simulink model "Final_simulation"  (R2024b)
settings: Solver=VariableStepAuto  StartTime=0  StopTime=5*4  FixedStep=1e-6  RelTol=1e-3
libraries: fl_lib x16, spsSeriesRLCBranchLib x9, nesl_utility x8, spsDiodeLib x6, spsMosfetLib x4, spsPWMGeneratorDCDCLib x4, spsControlledVoltageSourceLib x3, slpidlib x2, spsVoltageMeasurementLib x2, spsDCMachineLib x1, spsDCVoltageSourceLib x1, spsGroundLib x1
settings Model: SimulationMode=accelerator  Creator=06MBC93  LastModifiedBy=kamer
settings RTWCC: GPUComputeCapability=3.5

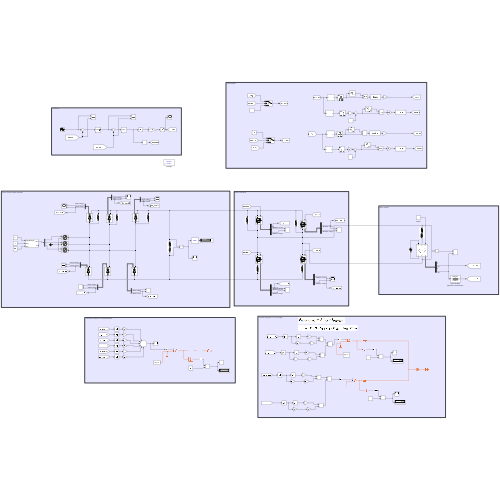
[thumbnail: Simulink's stored preview of the top-level diagram]
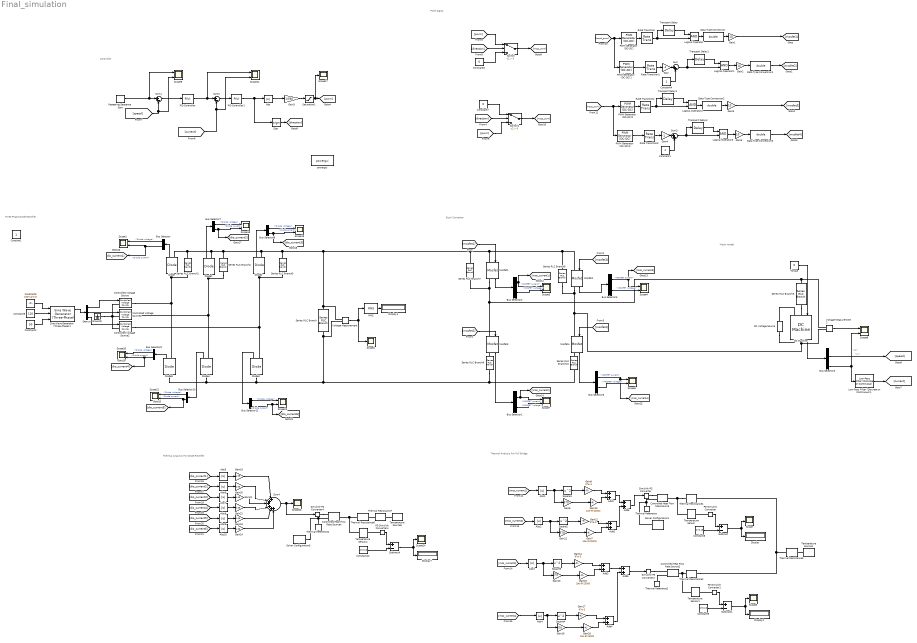
== system Final_simulation ==
  note: Thermal Analysis For Diode Rectifier
  note: Thermal Analysis For Full Bridge
  note: Three Phase Diode Rectifier
  note: Motor model
  note: Buck Converter
  note: PWM Signal
  note: Controller
  Abs{,1..10} (11 alike) : Abs  SaturateOnIntegerOverflow=off
  Add{1..6} (6 alike) : Sum
  Bus Selector{,7..11} (6 alike) : BusSelector  OutputSignals=Diode voltage,Diode current
  Bus Selector{1..2,5..6} (4 alike) : BusSelector  OutputSignals=MOSFET current,MOSFET voltage
  Bus Selector3 : BusSelector  OutputSignals=Te,w,iF,iA
  Constant1 : Constant
  Constant12 : Constant  Value=273.15
  Constant2 : Constant  Value=50
  Constant3 : Constant  Value=230*sqrt(2)
  Constant4 : Constant
  Constant5 : Constant  Value=120
  Constant6 : Constant  Value=0
  Constant7 : Constant  Value=0
  Constant8 : Constant  Value=273.15
  Constant9 : Constant  Value=273.15
  Controlled Heat Flow Rate Source : fl_lib/Thermal/Thermal Sources/Controlled Heat Flow Rate Source
  Controlled Heat Flow Rate Source2 : fl_lib/Thermal/Thermal Sources/Controlled Heat Flow Rate Source
  Controlled Heat Flow Rate Source4 : fl_lib/Thermal/Thermal Sources/Controlled Heat Flow Rate Source
  Controlled Voltage Source : spsControlledVoltageSourceLib/Controlled Voltage Source  Initialize=on  Source_Type=DC  Amplitude=0  Phase=0  Frequency=50  Measurements=None
  Controlled Voltage Source1 : spsControlledVoltageSourceLib/Controlled Voltage Source  Initialize=on  Source_Type=DC  Amplitude=0  Phase=120  Frequency=50  Measurements=None
  Controlled Voltage Source2 : spsControlledVoltageSourceLib/Controlled Voltage Source  Initialize=on  Source_Type=DC  Amplitude=0  Phase=240  Frequency=50  Measurements=None
  DC Machine : spsDCMachineLib/DC Machine  PresetModel=No  MechanicalLoad=Torque TL  FieldType=Wound  ShowDetailedParameters=on  MeasurementBus=on  RLa="[ 0.8  0.0125]"  RLf="[ 210  23]"  Laf=0.482  MachineConstant=Torque constant (N.m/A)  Ke=1.8  Kt=1.8  J=0.12  Bm=0.03  Tf=0.13  w0=0  Ifinit=1.04761904756944  TsPowergui=0  TsBlock=-1
  DC Voltage Source : spsDCVoltageSourceLib/DC Voltage Source  Amplitude=220  Measurements=None
  Data Type Conversion{,1..3} (4 alike) : DataTypeConversion  OutDataTypeStr=double  SaturateOnIntegerOverflow=off  RndMeth=Floor
  Demux : Demux  Outputs=3
  Diode{,1..5} (6 alike) : spsDiodeLib/Diode  Ron=0.015  Lon=0  Vf=1.05  IC=0  UseSnubber=0  Rs=inf  Cs=0  Measurements=on
  Display{,1..2,7} (4 alike) : Display
  Gain : Gain  Gain=-1
  Gain{1..2,5..6} (4 alike) : Gain  Gain=10
  Gain{7,10,15,18} (4 alike) : Gain  Gain=10e-9*25000
  Gain{8,11,13,16} (4 alike) : Gain  Gain=570
  Gain{9,12,14,17} (4 alike) : Gain  Gain=97e-3
  Gain{19..24} (6 alike) : Gain  Gain=1.05
  Gain3 : Gain  Gain=1/560
  Gain4 : Gain  Gain=-1
  Ground1 : spsGroundLib/Ground  LConnTagsString=a
  Logical Operator{,1..3} (4 alike) : Logic  AllPortsSameDT=off  OutDataTypeStr=boolean
  Low-Pass Filter (Discrete or Continuous)1 : eeGeneralControl/Low-Pass Filter (Discrete or Continuous)  K=1  T=0.008  B=inf  A=-inf  init_option=Inherited from block input  x0=0  Ts=-1
  Mosfet{1..4} (4 alike) : spsMosfetLib/Mosfet  Ron=97e-3*1.4  Lon=0  Rd=0.01  Vfd=1.6  IC=0  Rs=inf  Cs=0  Measurements=on
  PID Controller : slpidlib/PID Controller  Controller=PI  Form=Parallel  TimeDomain=Discrete-time  UseExternalTs=off  SampleTime=1/1000  IntegratorMethod=Forward Euler  FilterMethod=Forward Euler  ControllerParametersSource=internal  P=15  I=0.15  UseKiTs=on  D=0.001  UseExternalDerivativeSource=off  N=100  UseFilter=on  TunerSelectOption=Transfer Function Based (PID Tuner App)  InitialConditionSource=internal  InitialConditionForIntegrator=0  InitialConditionForFilter=0  DifferentiatorICPrevScaledInput=0  ExternalReset=none  TrackingMode=off  Kt=1  LimitOutput=on  SatLimitsSource=internal  UpperSaturationLimit=15  LowerSaturationLimit=-15  LinearizeAsGain=on  AntiWindupMode=clamping  Kb=1  LimitIntegrator=off  UpperIntegratorSaturationLimit=inf  LowerIntegratorSaturationLimit=-inf  POutMin=[]  POutMax=[]  IOutMin=[]  IOutMax=[]  DOutMin=[]  DOutMax=[]  NOutMin=[]  NOutMax=[]  SumOutMin=[]  SumOutMax=[]  SaturationOutMin=[]  SaturationOutMax=[]  PParamMin=[]  PParamMax=[]  IParamMin=[]  IParamMax=[]  DParamMin=[]  DParamMax=[]  NParamMin=[]  NParamMax=[]  KbParamMin=[]  KbParamMax=[]  KtParamMin=[]  KtParamMax=[]  KbOutMin=[]  KbOutMax=[]  KtOutMin=[]  KtOutMax=[]  IntegratorOutMin=[]  IntegratorOutMax=[]  FilterOutMin=[]  FilterOutMax=[]  SumI1OutMin=[]  SumI1OutMax=[]  SumI2OutMin=[]  SumI2OutMax=[]  SumI3OutMin=[]  SumI3OutMax=[]  SumI4OutMin=[]  SumI4OutMax=[]  SumDOutMin=[]  SumDOutMax=[]  DifferentiatorOutMin=[]  DifferentiatorOutMax=[]  FilterDiffOutCoefMin=[]  FilterDiffOutCoefMax=[]  ReciprocalOutMin=[]  ReciprocalOutMax=[]  SumDenOutMin=[]  SumDenOutMax=[]  SumNumOutMin=[]  SumNumOutMax=[]  DivideOutMin=[]  DivideOutMax=[]  UdiffTsProdOutMin=[]  UdiffTsProdOutMax=[]  NTsProdOutMin=[]  NTsProdOutMax=[]  UintegralTsProdOutMin=[]  UintegralTsProdOutMax=[]  UngainTsProdOutMin=[]  UngainTsProdOutMax=[]  ClampingZeroOutDataTypeStr=Inherit: Inherit via back propagation  ClampingZeroOutMin=[]  ClampingZeroOutMax=[]  FilterDenConstantOutDataTypeStr=Inherit: Inherit via back propagation  FilterDenConstantOutMin=[]  FilterDenConstantOutMax=[]  PCopyOutDataTypeStr=Inherit: Inherit via back propagation  PCopyOutMin=[]  PCopyOutMax=[]  NCopyOutDataTypeStr=Inherit: Inherit via back propagation  NCopyOutMin=[]  NCopyOutMax=[]  IntegratorContinuousStateAttributes=''  IntegratorStateMustResolveToSignalObject=off  IntegratorRTWStateStorageClass=Auto  FilterContinuousStateAttributes=''  FilterStateMustResolveToSignalObject=off  FilterRTWStateStorageClass=Auto  ParallelPVariant=InternalParameters  IdealPVariant=Disabled  IVariant=InternalParameters  DVariant=Disabled  IntegratorVariant=Discrete  SatVariant=Enabled  AWVariant=DiscClampingParallel  PCopyVariant=Disabled  TRVariant=Disabled  FdbkBlocksVariant=Forward  IdealPFdbkVariant=Disabled  SatFdbkVariant=Disabled  DerivativeFilterVariant=Disabled  NVariant=Disabled  NCopyVariant=Disabled_SignalSpec  FilterICVariant=Disabled  IntegratorICVariant=InternalICs  ExternalResetVariant=Disabled  TRSumVariant=Passthrough  SumFdbkVariant=Disabled  SumVariant=Sum_PI  TsampFilterVariant=InternalTs  TsampNgainVariant=Passthrough  TsampIntegralVariant=Disabled_SignalSpec  ExternalSaturationOutDataTypeStr=Inherit: Same as second input  DerivativeSourceVariant=Disabled  PreIntVariant=InternalPreInt
  PID Controller1 : slpidlib/PID Controller  Controller=PI  Form=Parallel  TimeDomain=Discrete-time  UseExternalTs=off  SampleTime=1/5000  IntegratorMethod=Forward Euler  FilterMethod=Forward Euler  ControllerParametersSource=internal  P=3  I=0.001  UseKiTs=on  D=0  UseExternalDerivativeSource=off  N=100  UseFilter=on  TunerSelectOption=Transfer Function Based (PID Tuner App)  InitialConditionSource=internal  InitialConditionForIntegrator=0  InitialConditionForFilter=0  DifferentiatorICPrevScaledInput=0  ExternalReset=none  TrackingMode=off  Kt=1  LimitOutput=off  SatLimitsSource=internal  UpperSaturationLimit=20  LowerSaturationLimit=-20  LinearizeAsGain=on  AntiWindupMode=clamping  Kb=1  LimitIntegrator=off  UpperIntegratorSaturationLimit=inf  LowerIntegratorSaturationLimit=-inf  POutMin=[]  POutMax=[]  IOutMin=[]  IOutMax=[]  DOutMin=[]  DOutMax=[]  NOutMin=[]  NOutMax=[]  SumOutMin=[]  SumOutMax=[]  SaturationOutMin=[]  SaturationOutMax=[]  PParamMin=[]  PParamMax=[]  IParamMin=[]  IParamMax=[]  DParamMin=[]  DParamMax=[]  NParamMin=[]  NParamMax=[]  KbParamMin=[]  KbParamMax=[]  KtParamMin=[]  KtParamMax=[]  KbOutMin=[]  KbOutMax=[]  KtOutMin=[]  KtOutMax=[]  IntegratorOutMin=[]  IntegratorOutMax=[]  FilterOutMin=[]  FilterOutMax=[]  SumI1OutMin=[]  SumI1OutMax=[]  SumI2OutMin=[]  SumI2OutMax=[]  SumI3OutMin=[]  SumI3OutMax=[]  SumI4OutMin=[]  SumI4OutMax=[]  SumDOutMin=[]  SumDOutMax=[]  DifferentiatorOutMin=[]  DifferentiatorOutMax=[]  FilterDiffOutCoefMin=[]  FilterDiffOutCoefMax=[]  ReciprocalOutMin=[]  ReciprocalOutMax=[]  SumDenOutMin=[]  SumDenOutMax=[]  SumNumOutMin=[]  SumNumOutMax=[]  DivideOutMin=[]  DivideOutMax=[]  UdiffTsProdOutMin=[]  UdiffTsProdOutMax=[]  NTsProdOutMin=[]  NTsProdOutMax=[]  UintegralTsProdOutMin=[]  UintegralTsProdOutMax=[]  UngainTsProdOutMin=[]  UngainTsProdOutMax=[]  ClampingZeroOutDataTypeStr=Inherit: Inherit via back propagation  ClampingZeroOutMin=[]  ClampingZeroOutMax=[]  FilterDenConstantOutDataTypeStr=Inherit: Inherit via back propagation  FilterDenConstantOutMin=[]  FilterDenConstantOutMax=[]  PCopyOutDataTypeStr=Inherit: Inherit via back propagation  PCopyOutMin=[]  PCopyOutMax=[]  NCopyOutDataTypeStr=Inherit: Inherit via back propagation  NCopyOutMin=[]  NCopyOutMax=[]  IntegratorContinuousStateAttributes=''  IntegratorStateMustResolveToSignalObject=off  IntegratorRTWStateStorageClass=Auto  FilterContinuousStateAttributes=''  FilterStateMustResolveToSignalObject=off  FilterRTWStateStorageClass=Auto  ParallelPVariant=InternalParameters  IdealPVariant=Disabled  IVariant=InternalParameters  DVariant=Disabled  IntegratorVariant=Discrete  SatVariant=Disabled  AWVariant=Passthrough  PCopyVariant=Disabled  TRVariant=Disabled  FdbkBlocksVariant=Forward  IdealPFdbkVariant=Disabled  SatFdbkVariant=Disabled  DerivativeFilterVariant=Disabled  NVariant=Disabled  NCopyVariant=Disabled_SignalSpec  FilterICVariant=Disabled  IntegratorICVariant=InternalICs  ExternalResetVariant=Disabled  TRSumVariant=Passthrough  SumFdbkVariant=Disabled  SumVariant=Sum_PI  TsampFilterVariant=InternalTs  TsampNgainVariant=Passthrough  TsampIntegralVariant=Disabled_SignalSpec  ExternalSaturationOutDataTypeStr=Inherit: Same as second input  DerivativeSourceVariant=Disabled  PreIntVariant=InternalPreInt
  PS-Simulink Converter : nesl_utility/PS-Simulink Converter  PhysicalDomain=network_engine_domain  SubClassName=ps_output  LeftPortType=input  RightPortType=output  PseudoPeriodic=off  Frequencies=[]  VectorFormat=inherit  Unit=degC  AffineConversion=off
  PS-Simulink Converter1 : nesl_utility/PS-Simulink Converter  PhysicalDomain=network_engine_domain  SubClassName=ps_output  LeftPortType=input  RightPortType=output  PseudoPeriodic=off  Frequencies=[]  VectorFormat=inherit  Unit=degC  AffineConversion=off
  PS-Simulink Converter4 : nesl_utility/PS-Simulink Converter  PhysicalDomain=network_engine_domain  SubClassName=ps_output  LeftPortType=input  RightPortType=output  PseudoPeriodic=off  Frequencies=[]  VectorFormat=inherit  Unit=degC  AffineConversion=off
  PWM Generator (DC-DC){,1..3} (4 alike) : spsPWMGeneratorDCDCLib/PWM Generator (DC-DC)  Fsw=25000  Ts=0
  RMS : spsRMSLib/RMS  TrueRMS=on  Freq=300  RMSInit=0  Ts=0
  Rate Transition{,1..3} (4 alike) : RateTransition  OutPortSampleTime=1e-6
  Repeating Sequence Stair : simulink/Sources/Repeating Sequence Stair  OutValues=[0 30 -30 0].'  tsamp=5  OutMin=[]  OutMax=[]  OutDataTypeStr=double  OutputDataTypeScalingMode=double  OutDataType=fixdt(0,8)  ConRadixGroup=Best Precision: Vector-wise  OutScaling=2^-12
  Saturation1 : Saturate  UpperLimit=0.32  LowerLimit=0
  Scope{,2,5,17,23..24} (6 alike) : Scope
  Scope{1,3..4,6..9,11,18..22} (13 alike) : Scope  NumInputPorts=2
  Series RLC Branch : spsSeriesRLCBranchLib/Series RLC Branch  LConnTagsString=__new0  RConnTagsString=__new0  BranchType=RC  Resistance=5.1e-3/2  Inductance=3e-3  SetiL0=off  InitialCurrent=0  Capacitance=100e-6*2  Setx0=on  InitialVoltage=561  Measurements=None
  Series RLC Branch{1..2,5,7..8} (5 alike) : spsSeriesRLCBranchLib/Series RLC Branch  LConnTagsString=__new0  RConnTagsString=__new0  BranchType=R  Resistance=1e11  Inductance=3e-3  SetiL0=off  InitialCurrent=0  Capacitance=100e-6*2  Setx0=on  InitialVoltage=565  Measurements=None
  Series RLC Branch10 : spsSeriesRLCBranchLib/Series RLC Branch  LConnTagsString=__new0  RConnTagsString=__new0  BranchType=R  Resistance=0.04  Inductance=3e-3  SetiL0=off  InitialCurrent=0  Capacitance=100e-6*2  Setx0=on  InitialVoltage=565  Measurements=None
  Series RLC Branch3 : spsSeriesRLCBranchLib/Series RLC Branch  LConnTagsString=__new0  RConnTagsString=__new0  BranchType=RL  Resistance=0.27  Inductance=12e-3  SetiL0=off  InitialCurrent=0  Capacitance=70e-6*4  Setx0=off  InitialVoltage=0  Measurements=None
  Series RLC Branch9 : spsSeriesRLCBranchLib/Series RLC Branch  LConnTagsString=__new0  RConnTagsString=__new0  BranchType=R  Resistance=0.04  Inductance=3e-3  SetiL0=off  InitialCurrent=0  Capacitance=100e-6*2  Setx0=on  InitialVoltage=565  Measurements=None
  Sign : Signum
  Simulink-PS Converter : nesl_utility/Simulink-PS Converter  PhysicalDomain=network_engine_domain  SubClassName=ps_input  LeftPortType=input  RightPortType=output  PseudoPeriodic=off  Frequencies=[]  NoiseDistribution=none  NoiseParameters=[]  Unit=1  AffineConversion=off  FilteringAndDerivatives=provide  SimscapeFilterOrder=1  InputFilterTimeConstant=0.001  UdotUserProvided=0
  Simulink-PS Converter2 : nesl_utility/Simulink-PS Converter  PhysicalDomain=network_engine_domain  SubClassName=ps_input  LeftPortType=input  RightPortType=output  PseudoPeriodic=off  Frequencies=[]  NoiseDistribution=none  NoiseParameters=[]  Unit=1  AffineConversion=off  FilteringAndDerivatives=provide  SimscapeFilterOrder=1  InputFilterTimeConstant=0.001  UdotUserProvided=0
  Simulink-PS Converter4 : nesl_utility/Simulink-PS Converter  PhysicalDomain=network_engine_domain  SubClassName=ps_input  LeftPortType=input  RightPortType=output  PseudoPeriodic=off  Frequencies=[]  NoiseDistribution=none  NoiseParameters=[]  Unit=1  AffineConversion=off  FilteringAndDerivatives=provide  SimscapeFilterOrder=1  InputFilterTimeConstant=0.001  UdotUserProvided=0
  Sine Wave Generator (Three-Phase)1 : eeSinGeneratorThreePhase/Sine Wave Generator (Three-Phase)  Ts=-1
      settings: LibrarySourceBlock=|
      | ee_sl_lib/General Control/Sine Wave Generator
      | (Three-Phase)
  Solver Configuration1 : nesl_utility/Solver Configuration  PhysicalDomain=network_engine_domain  SubClassName=solver  LeftPortType=input  RightPortType=generic  Tones=[]  Harmonics=[]  SimulateNoise=off  Profile=off  UseLocalSampling=off  EnableSwitchedLinearOptims=on  FrequencyDomain=off  UseCCode=off  RelTol=0.001  AbsTol=0.001  MinStep=1e-09  ToWorkspace=off  RevertToSquareIcSolve=off  NumHomotopyIterations=100  PhasorMode=off  PhasorModeNumHarmonics=1  ConsistencySolver=NEWTON_XTOL_AFTER_FTOL  IndexReductionMethod=DerivativeReplacement  DoDC=off  ResidualTolerance=1e-09  ConsistencyTolSource=GLOBAL  ConsistencyAbsTol=0.001  ConsistencyRelTol=0.001  ConsistencyTolFactor=0.001  UseLocalSolver=off  LocalSolverChoice=NE_BACKWARD_EULER_ADVANCER  ResolveIndetEquations=on  FunctionEvalNumThread=1  LocalSolverSampleTime=0.001  DoFixedCost=off  MaxNonlinIter=3  MaxModeIter=2  ComputeImpulses=off  ImpulseIterations=2  LinearAlgebra=auto  LinearAlgebraNumThread=0  EquationFormulation=NE_TIME_EF  DelaysMemoryBudget=1024  AutomaticFiltering=on  FilteringTimeConstant=0.001  PartitionStorageMethod=AS_NEEDED  PartitionMemoryBudget=1024  PartitionMethod=ROBUST  MultibodyUseLocalSolver=off  MultibodyLocalSolverChoice=ODE1  MultibodyLocalSolverSampleTime=0.001
  Solver Configuration5 : nesl_utility/Solver Configuration  PhysicalDomain=network_engine_domain  SubClassName=solver  LeftPortType=input  RightPortType=generic  Tones=[]  Harmonics=[]  SimulateNoise=off  Profile=off  UseLocalSampling=off  EnableSwitchedLinearOptims=on  FrequencyDomain=off  UseCCode=off  RelTol=0.001  AbsTol=0.001  MinStep=1e-09  ToWorkspace=off  RevertToSquareIcSolve=off  NumHomotopyIterations=100  PhasorMode=off  PhasorModeNumHarmonics=1  ConsistencySolver=NEWTON_XTOL_AFTER_FTOL  IndexReductionMethod=DerivativeReplacement  DoDC=off  ResidualTolerance=1e-09  ConsistencyTolSource=GLOBAL  ConsistencyAbsTol=0.001  ConsistencyRelTol=0.001  ConsistencyTolFactor=0.001  UseLocalSolver=off  LocalSolverChoice=NE_BACKWARD_EULER_ADVANCER  ResolveIndetEquations=on  FunctionEvalNumThread=1  LocalSolverSampleTime=0.001  DoFixedCost=off  MaxNonlinIter=3  MaxModeIter=2  ComputeImpulses=off  ImpulseIterations=2  LinearAlgebra=auto  LinearAlgebraNumThread=0  EquationFormulation=NE_TIME_EF  DelaysMemoryBudget=1024  AutomaticFiltering=on  FilteringTimeConstant=0.001  PartitionStorageMethod=AS_NEEDED  PartitionMemoryBudget=1024  PartitionMethod=ROBUST  MultibodyUseLocalSolver=off  MultibodyLocalSolverChoice=ODE1  MultibodyLocalSolverSampleTime=0.001
  Square{1..4} (4 alike) : Math  Operator=square
  Subtract : Sum  Inputs=+-
  Subtract1 : Sum  Inputs=+-
  Subtract4 : Sum  Inputs=+-
  Sum : Sum  Inputs=|++
  Sum1 : Sum  Inputs=|+-
  Sum2 : Sum  Inputs=|+-
  Sum3 : Sum  Inputs=|++
  Sum4 : Sum  Inputs=|++++++
  Switch : Switch  Criteria=u2 > Threshold  SaturateOnIntegerOverflow=off  InputSameDT=off
  Switch1 : Switch  Criteria=u2 > Threshold  SaturateOnIntegerOverflow=off  InputSameDT=off
  Temperature Sensor : fl_lib/Thermal/Thermal Sensors/Temperature Sensor  temperature_measure=foundation.enum.MeasurementReference.absolute
      settings: InternalSimscapePortConfiguration="{\"Bottom\":[],\"Left\":[{\"id\":\"A\",\"label\":\"A\",\"type\":\"foundation.thermal.thermal\"}],\"Right\":[{\"id\":\"T\",\"label\":\"T\",\"type\":\"output\"}],\"Top\":[]}"
  Temperature Sensor1 : fl_lib/Thermal/Thermal Sensors/Temperature Sensor  temperature_measure=foundation.enum.MeasurementReference.absolute
      settings: InternalSimscapePortConfiguration="{\"Bottom\":[],\"Left\":[{\"id\":\"A\",\"label\":\"A\",\"type\":\"foundation.thermal.thermal\"}],\"Right\":[{\"id\":\"T\",\"label\":\"T\",\"type\":\"output\"}],\"Top\":[]}"
  Temperature Sensor4 : fl_lib/Thermal/Thermal Sensors/Temperature Sensor  temperature_measure=foundation.enum.MeasurementReference.absolute
      settings: InternalSimscapePortConfiguration="{\"Bottom\":[],\"Left\":[{\"id\":\"A\",\"label\":\"A\",\"type\":\"foundation.thermal.thermal\"}],\"Right\":[{\"id\":\"T\",\"label\":\"T\",\"type\":\"output\"}],\"Top\":[]}"
  Temperature Source1 : fl_lib/Thermal/Thermal Sources/Temperature Source  temperature=25 degC
  Temperature Source5 : fl_lib/Thermal/Thermal Sources/Temperature Source  temperature=25 degC
  Thermal Reference : fl_lib/Thermal/Thermal Elements/Thermal Reference
  Thermal Reference2 : fl_lib/Thermal/Thermal Elements/Thermal Reference
  Thermal Reference4 : fl_lib/Thermal/Thermal Elements/Thermal Reference
  Thermal Resistance1 : fl_lib/Thermal/Thermal Elements/Thermal Resistance  resistance=0.6 K/W  T_specify=off  T_priority=None  T=0 K  T_nominal_specify=off  T_nominal_value=1  T_nominal_unit=K  Q_specify=off  Q_priority=None  Q=0 W  Q_nominal_specify=off  Q_nominal_value=1  Q_nominal_unit=W
  Thermal Resistance2 : fl_lib/Thermal/Thermal Elements/Thermal Resistance  resistance=0.6 K/W  T_specify=off  T_priority=None  T=0 K  T_nominal_specify=off  T_nominal_value=1  T_nominal_unit=K  Q_specify=off  Q_priority=None  Q=0 W  Q_nominal_specify=off  Q_nominal_value=1  Q_nominal_unit=W
  Thermal Resistance5 : fl_lib/Thermal/Thermal Elements/Thermal Resistance  resistance=0.47 K/W  T_specify=off  T_priority=None  T=0 K  T_nominal_specify=off  T_nominal_value=1  T_nominal_unit=K  Q_specify=off  Q_priority=None  Q=0 W  Q_nominal_specify=off  Q_nominal_value=1  Q_nominal_unit=W
  Thermal Resistance6 : fl_lib/Thermal/Thermal Elements/Thermal Resistance  resistance=1.8 K/W  T_specify=off  T_priority=None  T=0 K  T_nominal_specify=off  T_nominal_value=1  T_nominal_unit=K  Q_specify=off  Q_priority=None  Q=0 W  Q_nominal_specify=off  Q_nominal_value=1  Q_nominal_unit=W
  Thermal Resistance7 : fl_lib/Thermal/Thermal Elements/Thermal Resistance  resistance=0.5 K/W  T_specify=off  T_priority=None  T=0 K  T_nominal_specify=off  T_nominal_value=1  T_nominal_unit=K  Q_specify=off  Q_priority=None  Q=0 W  Q_nominal_specify=off  Q_nominal_value=1  Q_nominal_unit=W
  Torque : Constant  Value=0
  Transport Delay{,1..3} (4 alike) : TransportDelay  DelayTime=1/1000000  BufferSize=16384
  Voltage Measurement : spsVoltageMeasurementLib/Voltage Measurement  PhasorSimulation=off  OutputType=Complex  PSBequivalent=0
  Voltage Measurement2 : spsVoltageMeasurementLib/Voltage Measurement  PhasorSimulation=off  OutputType=Complex  PSBequivalent=0
  powergui : sps_lib/powergui  Priority=1  SimulationMode=Discrete  SampleTime=1e-6  frequency=60  Iterations=50  frequencyindice=0  Pbase=100e6  ErrMax=1e-4  UnitsV=kV  UnitsW=MW  buscounter=0  FunctionMessages=off  echomessages=off  EnableUseOfTLC=off  CurrentSourceSwitches=off  DisableSnubberDevices=off  DisableRonSwitches=off  DisableVfSwitches=off  DisplayEquations=off  AutomaticDiscreteSolvers=off  SolverType=Tustin/Backward Euler (TBE)  Interpol=off  ExternalGateDelay=off  methode=off  Ts=100  x0status=blocks  SPID=on  SwTol=0  HookPort=off  NonlinearTolerance=1e-4  nMaxIteration=100  ContinueOnMaxIteration=off  RestoreLinks=warning  ResistiveCurrentMeasurement=off  Frange=[0:2:500]  Ylog=off  Xlog=on  ShowGrid=off  save=off  variable=ZData  structure=0  ZoomFFT=off  StartTime=0.0  cycles=1  DisplayStyle=1  fundamental=60  FreqAxis=off  MaxFrequency=1000  frequencyindicesteady=1  RmsSteady=1  display=off
  Constan1 : Constant  IOType=siggen
  wires:
  Voltage Measurement/1 -> Scope2/1, RMS/1
  RMS/1 -> Display1/1
  Diode/1 -> Bus Selector/1
  Bus Selector/1 -> Scope1/1  "<Diode voltage>"
  Voltage Measurement2/1 -> Scope8/1
  [mosfet2] -> Mosfet3/1
  DC Machine/1 -> Bus Selector3/1
  Bus Selector3/4 -> Scope8/2, Low-Pass Filter (Discrete or Continuous)1/1  "<iA>"
  Constant4/1 -> Sum/2
  Gain/1 -> Sum/1
  Transport Delay/1 -> Logical Operator/1
  PWM Generator (DC-DC)/1 -> Rate Transition/1
  Sum/1 -> Logical Operator1/2, Transport Delay1/1
  Transport Delay1/1 -> Logical Operator1/1
  Logical Operator1/1 -> Gain2/1
  Logical Operator/1 -> Data Type Conversion/1
  Data Type Conversion/1 -> Gain1/1
  Data Type Conversion1/1 -> [mosfet2]
  [mosfet1] -> Mosfet1/1
  [mosfet3] -> Mosfet2/1
  [mosfet4] -> Mosfet4/1
  Gain2/1 -> Data Type Conversion1/1
  Gain1/1 -> [mosfet1]
  Rate Transition/1 -> Logical Operator/2, Transport Delay/1
  Rate Transition1/1 -> Gain/1
  [speed] -> Scope9/2, Sum1/2
  PID Controller/1 -> Scope11/1, Sum2/1
  [current] -> Scope11/2, Sum2/2
  Sum2/1 -> PID Controller1/1
  Sum1/1 -> PID Controller/1
  Gain5/1 -> [mosfet3]
  PWM Generator (DC-DC)1/1 -> Rate Transition1/1
  Bus Selector3/2 -> [speed]  "<w>"
  Torque/1 -> DC Machine/1
  PID Controller1/1 -> Sign/1, Abs/1
  Gain3/1 -> Saturation1/1
  Saturation1/1 -> Scope17/1, [pwm]
  [mos1_pwm] -> PWM Generator (DC-DC)1/1, PWM Generator (DC-DC)/1
  Constant5/1 -> Sine Wave Generator (Three-Phase)1/2
  Constant2/1 -> Sine Wave Generator (Three-Phase)1/3
  Sine Wave Generator (Three-Phase)1/1 -> Demux/1
  Demux/2 -> Controlled Voltage Source1/1
  Demux/3 -> Controlled Voltage Source2/1
  Demux/1 -> Controlled Voltage Source/1
  Mosfet3/1 -> Bus Selector1/1
  Mosfet2/1 -> Bus Selector5/1
  Mosfet1/1 -> Bus Selector2/1
  Mosfet4/1 -> Bus Selector6/1
  Bus Selector2/2 -> Scope3/2  "<MOSFET voltage>"
  Bus Selector5/1 -> [mos_current3], Scope4/1  "<MOSFET current>"
  Bus Selector5/2 -> Scope4/2  "<MOSFET voltage>"
  Bus Selector6/1 -> [mos_current4], Scope6/1  "<MOSFET current>"
  Bus Selector6/2 -> Scope6/2  "<MOSFET voltage>"
  Bus Selector1/2 -> Scope7/2  "<MOSFET voltage>"
  Low-Pass Filter (Discrete or Continuous)1/1 -> [current]
  Sign/1 -> [direction]
  [direction] -> Switch/2
  [pwm] -> Switch/1
  Constant6/1 -> Switch/3
  Switch/1 -> [mos1_pwm]
  Switch1/1 -> [mos2_pwm]
  Constant7/1 -> Switch1/1
  [pwm] -> Switch1/3
  [direction] -> Switch1/2
  [mos2_pwm] -> PWM Generator (DC-DC)2/1, PWM Generator (DC-DC)3/1
  PWM Generator (DC-DC)3/1 -> Rate Transition3/1
  Rate Transition3/1 -> Gain4/1
  Rate Transition2/1 -> Transport Delay2/1, Logical Operator2/2
  Gain6/1 -> Data Type Conversion3/1
  Data Type Conversion3/1 -> [mosfet4]
  Data Type Conversion2/1 -> Gain5/1
  Logical Operator2/1 -> Data Type Conversion2/1
  Logical Operator3/1 -> Gain6/1
  Transport Delay3/1 -> Logical Operator3/1
  Sum3/1 -> Transport Delay3/1, Logical Operator3/2
  PWM Generator (DC-DC)2/1 -> Rate Transition2/1
  Transport Delay2/1 -> Logical Operator2/1
  Gain4/1 -> Sum3/1
  Constant1/1 -> Sum3/2
  Abs/1 -> Gain3/1
  Constant3/1 -> Sine Wave Generator (Three-Phase)1/1
  PS-Simulink Converter/1 -> Subtract/1
  Constant8/1 -> Subtract/2
  Subtract/1 -> Display/1, Scope/1
  Gain9/1 -> Add1/1
  Square1/1 -> Gain9/1
  Gain8/1 -> Gain10/1
  Gain10/1 -> Add1/2
  [mos_current1] -> Abs1/1
  Add1/1 -> Add5/1
  Add2/1 -> Add5/2
  [mos_current2] -> Abs2/1
  Gain7/1 -> Add2/2
  Gain11/1 -> Gain7/1
  Square2/1 -> Gain12/1
  Gain12/1 -> Add2/1
  Gain14/1 -> Add3/1
  Square3/1 -> Gain14/1
  Gain13/1 -> Gain15/1
  Gain15/1 -> Add3/2
  [mos_current3] -> Abs3/1
  [mos_current4] -> Abs4/1
  Gain18/1 -> Add4/2
  Gain16/1 -> Gain18/1
  Square4/1 -> Gain17/1
  Gain17/1 -> Add4/1
  Add5/1 -> Simulink-PS Converter/1
  Bus Selector7/1 -> Scope18/1  "<Diode voltage>"
  Bus Selector7/2 -> [dio_current2], Scope18/2  "<Diode current>"
  Diode1/1 -> Bus Selector7/1
  Bus Selector8/2 -> [dio_current3], Scope19/2  "<Diode current>"
  Bus Selector8/1 -> Scope19/1  "<Diode voltage>"
  Diode2/1 -> Bus Selector8/1
  Bus Selector9/2 -> [dio_current4], Scope20/2  "<Diode current>"
  Bus Selector9/1 -> Scope20/1  "<Diode voltage>"
  Diode5/1 -> Bus Selector9/1
  Bus Selector10/1 -> Scope21/1  "<Diode voltage>"
  Bus Selector10/2 -> [dio_current5], Scope21/2  "<Diode current>"
  Diode4/1 -> Bus Selector10/1
  Bus Selector11/2 -> [dio_current6], Scope22/2  "<Diode current>"
  Bus Selector11/1 -> Scope22/1  "<Diode voltage>"
  Diode3/1 -> Bus Selector11/1
  [dio_current1] -> Abs5/1
  [dio_current2] -> Abs6/1
  [dio_current3] -> Abs7/1
  [dio_current4] -> Abs8/1
  [dio_current5] -> Abs9/1
  [dio_current6] -> Abs10/1
  Gain19/1 -> Sum4/1
  Gain20/1 -> Sum4/2
  Gain21/1 -> Sum4/3
  Gain22/1 -> Sum4/4
  Gain23/1 -> Sum4/5
  Gain24/1 -> Sum4/6
  Abs1/1 -> Gain8/1, Square1/1
  Abs2/1 -> Square2/1, Gain11/1
  Abs3/1 -> Gain13/1, Square3/1
  Abs4/1 -> Square4/1, Gain16/1
  Abs5/1 -> Gain19/1
  Abs6/1 -> Gain20/1
  Abs7/1 -> Gain21/1
  Abs8/1 -> Gain22/1
  Abs9/1 -> Gain23/1
  Abs10/1 -> Gain24/1
  Sum4/1 -> Scope23/1, Simulink-PS Converter4/1
  Subtract4/1 -> Scope24/1, Display7/1
  Constant12/1 -> Subtract4/2
  PS-Simulink Converter4/1 -> Subtract4/1
  Bus Selector/2 -> [dio_current1], Scope1/2  "<Diode current>"
  Bus Selector2/1 -> [mos_current1], Scope3/1  "<MOSFET current>"
  Bus Selector1/1 -> [mos_current2], Scope7/1  "<MOSFET current>"
  Add3/1 -> Add6/1
  Add4/1 -> Add6/2
  Add6/1 -> Simulink-PS Converter2/1
  Subtract1/1 -> Scope5/1, Display2/1
  Constant9/1 -> Subtract1/2
  PS-Simulink Converter1/1 -> Subtract1/1
  Repeating Sequence Stair/1 -> Scope9/1, Sum1/1
  connections:
  Diode2/LConn1 -- Controlled Voltage Source2/RConn1 -- Diode3/RConn1 -- Series RLC Branch5/RConn1
  Mosfet1/RConn1 -- Voltage Measurement2/LConn1 -- Series RLC Branch3/LConn1 -- Mosfet3/LConn1 -- Series RLC Branch7/RConn1
  Mosfet4/LConn1 -- DC Machine/RConn1 -- Voltage Measurement2/LConn2 -- Mosfet2/RConn1 -- Series RLC Branch8/RConn1
  DC Voltage Source/LConn1 -- DC Machine/RConn2
  DC Machine/LConn2 -- DC Voltage Source/RConn1
  Series RLC Branch3/RConn1 -- DC Machine/LConn1
  Diode5/RConn1 -- Series RLC Branch1/RConn1 -- Diode/LConn1 -- Controlled Voltage Source/RConn1
  Diode1/LConn1 -- Controlled Voltage Source1/RConn1 -- Diode4/RConn1 -- Series RLC Branch2/RConn1
  Ground1/LConn1 -- Controlled Voltage Source2/LConn1 -- Controlled Voltage Source1/LConn1 -- Controlled Voltage Source/LConn1
  Thermal Resistance1/LConn1 -- Controlled Heat Flow Rate Source/LConn1 -- Temperature Sensor/LConn1
  Thermal Reference/LConn1 -- Solver Configuration1/RConn1 -- Controlled Heat Flow Rate Source/RConn2
  Thermal Resistance5/LConn1 -- Thermal Resistance2/RConn1 -- Thermal Resistance1/RConn1
  PS-Simulink Converter/LConn1 -- Temperature Sensor/RConn1
  Simulink-PS Converter/RConn1 -- Controlled Heat Flow Rate Source/RConn1
  Thermal Resistance2/LConn1 -- Temperature Sensor1/LConn1 -- Controlled Heat Flow Rate Source2/LConn1
  Thermal Reference2/LConn1 -- Controlled Heat Flow Rate Source2/RConn2
  Simulink-PS Converter2/RConn1 -- Controlled Heat Flow Rate Source2/RConn1
  Temperature Source1/LConn1 -- Thermal Resistance5/RConn1
  Controlled Heat Flow Rate Source4/LConn1 -- Thermal Resistance6/LConn1 -- Temperature Sensor4/LConn1
  Solver Configuration5/RConn1 -- Thermal Reference4/LConn1 -- Controlled Heat Flow Rate Source4/RConn2
  Simulink-PS Converter4/RConn1 -- Controlled Heat Flow Rate Source4/RConn1
  Temperature Source5/LConn1 -- Thermal Resistance7/RConn1
  PS-Simulink Converter4/LConn1 -- Temperature Sensor4/RConn1
  Thermal Resistance7/LConn1 -- Thermal Resistance6/RConn1
  Mosfet3/RConn1 -- Series RLC Branch9/LConn1
  Series RLC Branch10/LConn1 -- Mosfet4/RConn1
  PS-Simulink Converter1/LConn1 -- Temperature Sensor1/RConn1
  Diode3/LConn1 -- Diode5/LConn1 -- Diode4/LConn1 -- Series RLC Branch10/RConn1 -- Series RLC Branch9/RConn1 -- Series RLC Branch/RConn1 -- Voltage Measurement/LConn2
  Diode/RConn1 -- Series RLC Branch5/LConn1 -- Mosfet2/LConn1 -- Series RLC Branch8/LConn1 -- Mosfet1/LConn1 -- Series RLC Branch7/LConn1 -- Voltage Measurement/LConn1 -- Series RLC Branch/LConn1 -- Diode2/RConn1 -- Series RLC Branch2/LConn1 -- Diode1/RConn1 -- Series RLC Branch1/LConn1
